simulink model "quadReduced"  (R2024a)
settings: Solver=VariableStepAuto  StartTime=0.0  StopTime=20  RelTol=1e-3
values from neighbouring files (symbols this model uses):
  A_x = 0.25    [playgrounMat.m]    (also in start.m; startEnglPaper.m; startReduced.m)
  A_y = 0.25    [playgrounMat.m]    (also in start.m; startEnglPaper.m; startReduced.m)
  A_z = 0.25    [playgrounMat.m]    (also in start.m; startEnglPaper.m; startReduced.m)
  b = 1.14 * 10^(-7)    (= 1.14e-07)    [start.m]    (also in startEnglPaper.m = 0.033)
  dt = 1e-4    (= 0.0001)    [start.m]    (also in startReduced.m)
  g = 9.81    [playgrounMat.m]    (also in start.m; startEnglPaper.m; startReduced.m)
  gamma_d = pi/3    (= 1.0471975512)    [start.m]    (also in startReduced.m = 0.2)
  I_r = 5.38 * 10 ^ (-5)    (= 5.38e-05)    [start.m]    (also in startEnglPaper.m = 3.38e-05; startReduced.m)
  I_x = 0.0151    [start.m]    (also in startEnglPaper.m = 0.004856; startReduced.m)
  I_y = 0.253    [start.m]    (also in startEnglPaper.m = 0.004856; startReduced.m = 0.0253)
  I_z = 0.0151    [start.m]    (also in startEnglPaper.m = 0.008801; startReduced.m)
  Icm = diag([Ix Iy Iz])    [start.m]    (also in startReduced.m)
  initial_quaternion = quaternion(initial_angles, 'euler', 'ZYX', 'frame')    [start.m]    (also in startReduced.m)
  k = 1.045 * 10^(-11)    (= 1.045e-11)    [start.m]    (also in startEnglPaper.m = 2.98e-06)
  K_gamma_D = 50    [start.m]    (also in startReduced.m = 0.14)
  K_gamma_D1 = K(1)    [playgrounMat.m]    (also in startReduced.m = 0.28992)
  K_gamma_I1 = K(3)    [playgrounMat.m]    (also in startReduced.m = 3.9584)
  K_gamma_P = 108    [start.m]    (also in startReduced.m = 0.35)
  K_gamma_P1 = K(2)    [playgrounMat.m]    (also in startReduced.m = 1.85548)
  K_psi_D = 40    [start.m]    (also in startEnglPaper.m = 9.6; startReduced.m = 0.24)
  K_psi_D1 = 0.0844    [startEnglPaper.m]    (also in startReduced.m = 0.4858)
  K_psi_I1 = 0    [startEnglPaper.m]    (also in startReduced.m = 6.6322)
  K_psi_P = 143    [start.m]    (also in startEnglPaper.m = 23.04; startReduced.m = 0.58)
  K_psi_P1 = 0.202    [startEnglPaper.m]    (also in startReduced.m = 3.11)
  K_theta_D = 58    [start.m]    (also in startEnglPaper.m = 9.6; startReduced.m = 0.14)
  K_theta_P = 141    [start.m]    (also in startEnglPaper.m = 23.04; startReduced.m = 0.35)
  K_y_D = 13.58    [start.m]    (also in startReduced.m)
  K_y_P = 33.18    [start.m]    (also in startReduced.m)
  l = 0.225    [start.m]    (also in startEnglPaper.m; startReduced.m)
  m = 1.44    [playgrounMat.m]    (also in start.m; startEnglPaper.m = 0.486; startReduced.m)
  m_s = [1/4 0 -1/(2*l) -1/(4*a_r); 1/4 -1/(2*l) 0 1/(4*a_r); 1/4 0 1/(2*l) -1/(4*a_r); 1/4 1/(2*l) 0 1/(4*a_r)]    [start.m]    (also in startReduced.m)
  omega_r = 1    [start.m]    (also in startReduced.m = 4)
  P_omega = diag([P_omega_x P_omega_y P_omega_z])    [start.m]    (also in startReduced.m)
  P_q = diag([P_q1 P_q2 P_q3])    [start.m]    (also in startReduced.m)
  psi_d = pi/5    (= 0.628318530718)    [start.m]    (also in startEnglPaper.m = 0.1; startReduced.m = 0.1)
  task_quaternion = quaternion(task_angles, 'euler', 'ZYX', 'frame')    [start.m]    (also in startReduced.m)
  theta_d = pi/4    (= 0.785398163397)    [start.m]    (also in startEnglPaper.m = -0.1; startReduced.m = -0.1)
  y_d = 100    [start.m]    (also in startReduced.m = 0.2)
undefined symbols (not defined in the file or in its folder): compact
libraries: slpidlib x4, aerolibutil x2, sharedtransform x1
(part 1 of 2)
settings Model: Creator=Оздоев  LastModifiedBy=Илья
settings SolverCC: ZeroCrossAlgorithm=Adaptive  AlgebraicLoopSolver=TrustRegion
settings DebuggingCC: IgnoredZcDiagnostic=none  UnconnectedInputMsg=warning  UnconnectedOutputMsg=warning  UnconnectedLineMsg=warning  ArithmeticOperatorsInVariantConditions=warning
settings ModelReferenceCC: EnableRefExpFcnMdlSchedulingChecks=on
settings SFSimCC: CustomCodeUndefinedFunction=UseInterfaceOnly
settings RTWCC: GPUComputeCapability=3.5

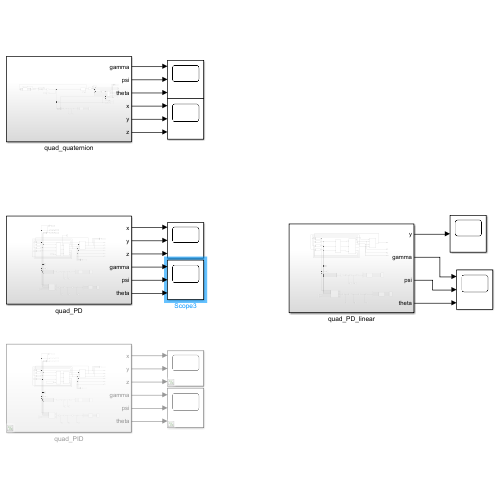
[thumbnail: Simulink's stored preview of the top-level diagram]
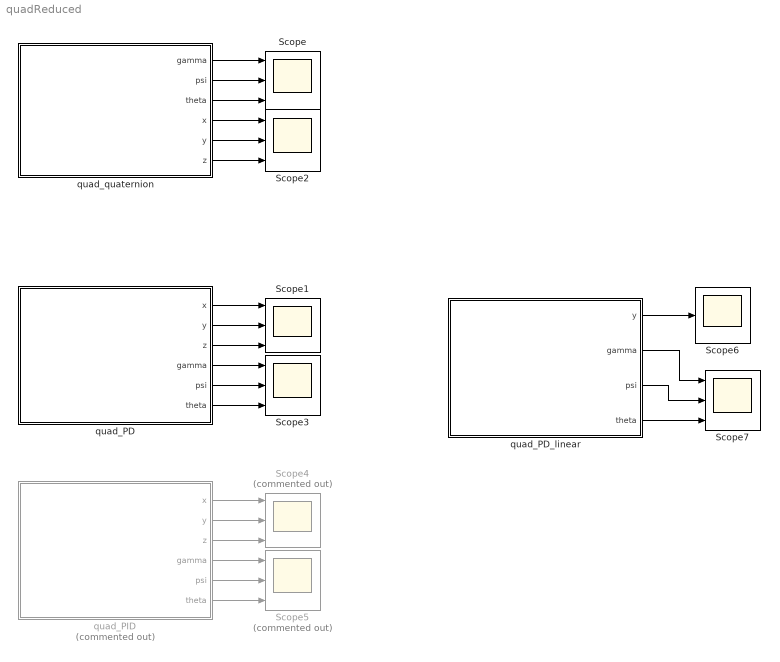
== system quadReduced ==
  Scope{,1..3,7} (5 alike) : Scope  NumInputPorts=3
  Scope4 : Scope  Commented=on  NumInputPorts=3
  Scope5 : Scope  Commented=on  NumInputPorts=3
  Scope6 : Scope
  quad_PD : Subsystem
  quad_PD_linear : Subsystem
  quad_PID : Subsystem  Commented=on
  quad_quaternion : Subsystem
  wires:
  quad_quaternion/1(gamma) -> Scope/1
  quad_quaternion/2(psi) -> Scope/2
  quad_quaternion/3(theta) -> Scope/3
  quad_quaternion/4(x) -> Scope2/1
  quad_quaternion/5(y) -> Scope2/2
  quad_quaternion/6(z) -> Scope2/3
  quad_PD/1(x) -> Scope1/1
  quad_PD/2(y) -> Scope1/2
  quad_PD/3(z) -> Scope1/3
  quad_PD/4(gamma) -> Scope3/1
  quad_PD/5(psi) -> Scope3/2
  quad_PD/6(theta) -> Scope3/3
  quad_PID/6(theta) -> Scope5/3
  quad_PID/5(psi) -> Scope5/2
  quad_PID/4(gamma) -> Scope5/1
  quad_PID/3(z) -> Scope4/3
  quad_PID/2(y) -> Scope4/2
  quad_PID/1(x) -> Scope4/1
  quad_PD_linear/4(theta) -> Scope7/3
  quad_PD_linear/3(psi) -> Scope7/2
  quad_PD_linear/2(gamma) -> Scope7/1
  quad_PD_linear/1(y) -> Scope6/1

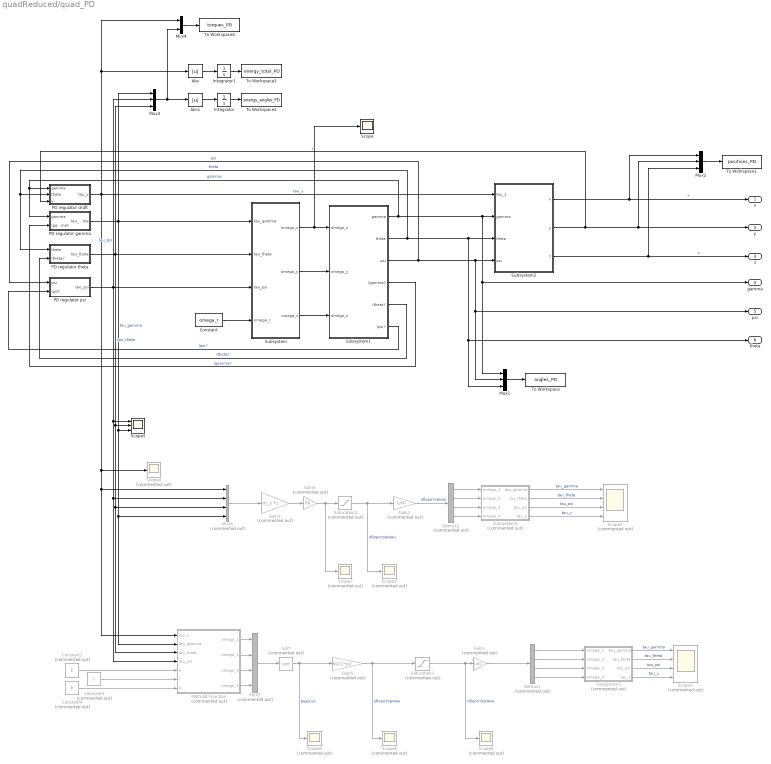
== system quadReduced/quad_PD ==
  Abs : Abs  SaturateOnIntegerOverflow=off
  Abs1 : Abs  SaturateOnIntegerOverflow=off
  Constant : Constant  Value=omega_r
  Constant2 : Constant  Commented=on  Value=k
  Constant3 : Constant  Commented=on  Value=l
  Constant4 : Constant  Commented=on  Value=b
  Demux1 : Demux  Commented=on
  Demux2 : Demux  Commented=on
  Gain1 : Gain  Commented=on  Gain=1/60
  Gain2 : Gain  Commented=on  Gain=1/60
  Gain3 : Gain  Commented=on  Gain=m_s  Multiplication=Matrix(K*u) (u vector)
  Gain5 : Gain  Commented=on  Gain=60/(2*pi)
  Gain6 : Gain  Commented=on  Gain=60
  Integrator : Integrator
  Integrator1 : Integrator
  MATLAB Function : MATLAB Function  Commented=on  TreatAsAtomicUnit=on
  Mux1 : Mux  Inputs=3
  Mux2 : Mux  Inputs=3
  Mux3 : Mux  Inputs=3
  Mux4 : Mux  Inputs=2
  Mux5 : Mux  Commented=on
  Mux6 : Mux  Commented=on
  PD regulator draft : Subsystem
  PD regulator gamma : Subsystem
  PD regulator psi : Subsystem
  PD regulator theta : Subsystem
  Saturation1 : Saturate  Commented=on  UpperLimit=15000  LowerLimit=1000
  Saturation2 : Saturate  Commented=on  UpperLimit=15000  LowerLimit=1000
  Scope : Scope
  Scope1 : Scope  Commented=on  NumInputPorts=4
  Scope{2,4,6..9} (6 alike) : Scope  Commented=on
  Scope3 : Scope  Commented=on  NumInputPorts=4
  Scope5 : Scope  NumInputPorts=3
  Sqrt : Sqrt  Commented=on
  Subsystem : Subsystem
  Subsystem1 : Subsystem
  Subsystem2 : Subsystem
  Subsystem3 : Subsystem  Commented=on
  Subsystem4 : Subsystem  Commented=on
  To Workspace : ToWorkspace  VariableName=angles_PD  SaveFormat=Structure With Time  SampleTime=-1
  To Workspace1 : ToWorkspace  VariableName=positions_PD  SaveFormat=Structure With Time  SampleTime=-1
  To Workspace2 : ToWorkspace  VariableName=energy_angles_PD  SaveFormat=Structure With Time  SampleTime=-1
  To Workspace3 : ToWorkspace  VariableName=energy_total_PD  SaveFormat=Structure With Time  SampleTime=-1
  To Workspace4 : ToWorkspace  VariableName=torques_PD  SaveFormat=Structure With Time  SampleTime=-1
  x : Outport
  y : Outport  Port=2
  z : Outport  Port=3
  gamma : Outport  Port=4
  psi : Outport  Port=5
  theta : Outport  Port=6
  wires:
  Subsystem1/1(gamma) -> gamma/1, Mux1/1, Subsystem2/2(gamma), PD regulator gamma/1(gamma), PD regulator draft/1(gamma)  "gamma"
  Subsystem/2(omega_y) -> Subsystem1/2(omega_y)
  Subsystem/3(omega_z) -> Subsystem1/3(omega_z)
  PD regulator theta/1(tau_theta) -> Subsystem/2(tau_theta), MATLAB Function/3(tau_theta), Mux6/3, Scope5/2, Mux3/3  "tau_theta"
  Mux1/1 -> To Workspace/1
  Subsystem1/5((theta)') -> PD regulator theta/2((theta)')  "(theta)'"
  Constant/1 -> Subsystem/4(omega_r)
  Subsystem/1(omega_x) -> Scope/1, Subsystem1/1(omega_x)
  Subsystem2/1(x) -> Mux2/1, x/1  "x"
  PD regulator gamma/1(tau_gamma) -> Subsystem/1(tau_gamma), Mux3/1, MATLAB Function/2(tau_gamma), Mux6/4, Scope5/3  "tau_gamma"
  Subsystem2/2(y) -> Mux2/2, y/1, PD regulator draft/3(y)  "y"
  Subsystem1/4((gamma)') -> PD regulator gamma/2((gamma)')  "(gamma)'"
  PD regulator psi/1(tau_psi) -> Subsystem/3(tau_psi), Mux3/2, MATLAB Function/4(tau_psi), Mux6/2, Scope5/1  "tau_psi"
  Subsystem1/3(psi) -> psi/1, Mux1/2, Subsystem2/4(psi), PD regulator psi/1(psi)  "psi"
  Subsystem1/6((psi)') -> PD regulator psi/2((psi)')  "(psi)'"
  Subsystem1/2(theta) -> Subsystem2/3(theta), theta/1, Mux1/3, PD regulator theta/1(theta), PD regulator draft/2(theta)  "theta"
  Subsystem2/3(z) -> Mux2/3, z/1  "z"
  Mux2/1 -> To Workspace1/1
  Integrator/1 -> To Workspace2/1
  Mux3/1 -> Mux4/2, Abs1/1
  Integrator1/1 -> To Workspace3/1
  Abs/1 -> Integrator1/1
  Abs1/1 -> Integrator/1
  Mux4/1 -> To Workspace4/1
  Subsystem3/2(tau_theta) -> Scope1/2  "tau_theta"
  Subsystem3/3(tau_psi) -> Scope1/3  "tau_psi"
  Subsystem3/1(tau_gamma) -> Scope1/1  "tau_gamma"
  Constant2/1 -> MATLAB Function/5(k)
  Constant3/1 -> MATLAB Function/6(l)
  Constant4/1 -> MATLAB Function/7(b)
  MATLAB Function/1(omega_1) -> Mux5/1
  MATLAB Function/2(omega_2) -> Mux5/2
  MATLAB Function/3(omega_3) -> Mux5/3
  MATLAB Function/4(omega_4) -> Mux5/4
  Mux5/1 -> Sqrt/1
  PD regulator draft/1(tau_y) -> Subsystem2/1(tau_y), Abs/1, Mux4/1, MATLAB Function/1(tau_y), Mux6/1, Scope4/1  "tau_y"
  Subsystem3/4(tau_y) -> Scope1/4  "tau_y"
  Mux6/1 -> Gain3/1
  Subsystem4/2(tau_theta) -> Scope3/2  "tau_theta"
  Subsystem4/3(tau_psi) -> Scope3/3  "tau_psi"
  Demux2/2 -> Subsystem4/2(omega_2)
  Demux2/1 -> Subsystem4/1(omega_1)
  Demux2/4 -> Subsystem4/4(omega_4)
  Demux2/3 -> Subsystem4/3(omega_3)
  Subsystem4/4(tau_y) -> Scope3/4  "tau_y"
  Subsystem4/1(tau_gamma) -> Scope3/1  "tau_gamma"
  Demux1/3 -> Subsystem3/3(omega_3)
  Demux1/4 -> Subsystem3/4(omega_4)
  Demux1/1 -> Subsystem3/1(omega_1)
  Demux1/2 -> Subsystem3/2(omega_2)
  Saturation2/1 -> Gain2/1, Scope2/1  "оборотов/мин"
  Gain6/1 -> Scope7/1, Saturation2/1
  Sqrt/1 -> Scope9/1, Gain5/1  "рад/сек"
  Saturation1/1 -> Gain1/1, Scope6/1  "оборотов/мин"
  Gain3/1 -> Gain6/1
  Gain5/1 -> Saturation1/1, Scope8/1  "оборотов/мин"
  Gain1/1 -> Demux1/1
  Gain2/1 -> Demux2/1  "оборотов/сек"

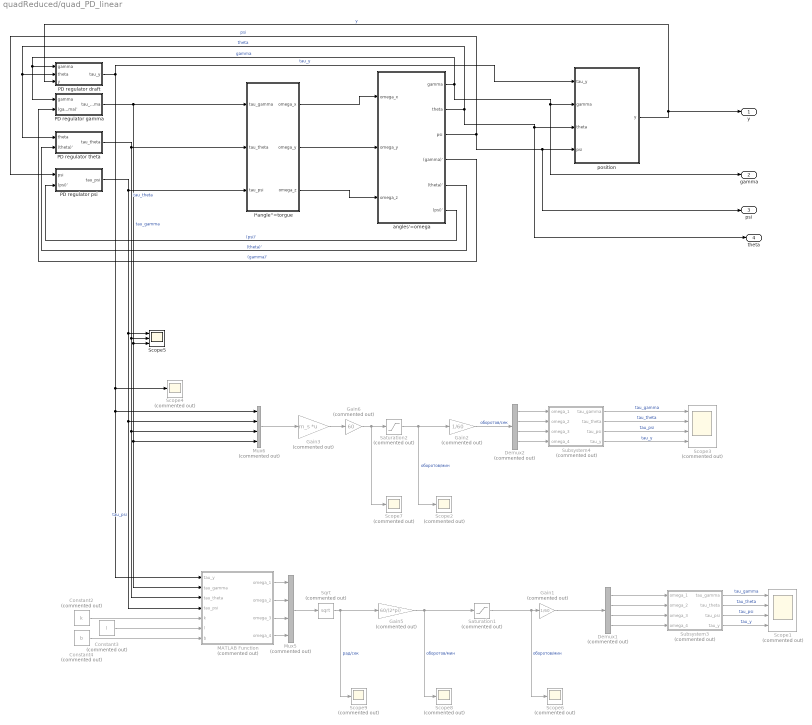
== system quadReduced/quad_PD_linear ==
  Constant2 : Constant  Commented=on  Value=k
  Constant3 : Constant  Commented=on  Value=l
  Constant4 : Constant  Commented=on  Value=b
  Demux1 : Demux  Commented=on
  Demux2 : Demux  Commented=on
  Gain1 : Gain  Commented=on  Gain=1/60
  Gain2 : Gain  Commented=on  Gain=1/60
  Gain3 : Gain  Commented=on  Gain=m_s  Multiplication=Matrix(K*u) (u vector)
  Gain5 : Gain  Commented=on  Gain=60/(2*pi)
  Gain6 : Gain  Commented=on  Gain=60
  I*angle''=torgue : Subsystem
  MATLAB Function : MATLAB Function  Commented=on  TreatAsAtomicUnit=on
  Mux5 : Mux  Commented=on
  Mux6 : Mux  Commented=on
  PD regulator draft : Subsystem
  PD regulator gamma : Subsystem
  PD regulator psi : Subsystem
  PD regulator theta : Subsystem
  Saturation1 : Saturate  Commented=on  UpperLimit=15000  LowerLimit=1000
  Saturation2 : Saturate  Commented=on  UpperLimit=15000  LowerLimit=1000
  Scope1 : Scope  Commented=on  NumInputPorts=4
  Scope{2,4,6..9} (6 alike) : Scope  Commented=on
  Scope3 : Scope  Commented=on  NumInputPorts=4
  Scope5 : Scope  NumInputPorts=3
  Sqrt : Sqrt  Commented=on
  Subsystem3 : Subsystem  Commented=on
  Subsystem4 : Subsystem  Commented=on
  angles'=omega : Subsystem
  position : Subsystem
  y : Outport
  gamma : Outport  Port=2
  psi : Outport  Port=3
  theta : Outport  Port=4
  wires:
  Gain2/1 -> Demux2/1  "оборотов/сек"
  Gain1/1 -> Demux1/1
  Gain5/1 -> Scope8/1, Saturation1/1  "оборотов/мин"
  Gain3/1 -> Gain6/1
  Saturation1/1 -> Scope6/1, Gain1/1  "оборотов/мин"
  Sqrt/1 -> Gain5/1, Scope9/1  "рад/сек"
  Gain6/1 -> Saturation2/1, Scope7/1
  Saturation2/1 -> Scope2/1, Gain2/1  "оборотов/мин"
  Demux1/2 -> Subsystem3/2(omega_2)
  Demux1/1 -> Subsystem3/1(omega_1)
  Demux1/4 -> Subsystem3/4(omega_4)
  Demux1/3 -> Subsystem3/3(omega_3)
  Subsystem4/1(tau_gamma) -> Scope3/1  "tau_gamma"
  Subsystem4/4(tau_y) -> Scope3/4  "tau_y"
  Demux2/3 -> Subsystem4/3(omega_3)
  Demux2/4 -> Subsystem4/4(omega_4)
  Demux2/1 -> Subsystem4/1(omega_1)
  Demux2/2 -> Subsystem4/2(omega_2)
  Subsystem4/3(tau_psi) -> Scope3/3  "tau_psi"
  Subsystem4/2(tau_theta) -> Scope3/2  "tau_theta"
  Mux6/1 -> Gain3/1
  Subsystem3/4(tau_y) -> Scope1/4  "tau_y"
  PD regulator draft/1(tau_y) -> Scope4/1, Mux6/1, MATLAB Function/1(tau_y), position/1(tau_y)  "tau_y"
  Mux5/1 -> Sqrt/1
  MATLAB Function/4(omega_4) -> Mux5/4
  MATLAB Function/3(omega_3) -> Mux5/3
  MATLAB Function/2(omega_2) -> Mux5/2
  MATLAB Function/1(omega_1) -> Mux5/1
  Constant4/1 -> MATLAB Function/7(b)
  Constant3/1 -> MATLAB Function/6(l)
  Constant2/1 -> MATLAB Function/5(k)
  Subsystem3/1(tau_gamma) -> Scope1/1  "tau_gamma"
  Subsystem3/3(tau_psi) -> Scope1/3  "tau_psi"
  Subsystem3/2(tau_theta) -> Scope1/2  "tau_theta"
  angles'=omega/2(theta) -> theta/1, position/3(theta), PD regulator draft/2(theta), PD regulator theta/1(theta)  "theta"
  angles'=omega/6((psi)') -> PD regulator psi/2((psi)')  "(psi)'"
  angles'=omega/3(psi) -> position/4(psi), psi/1, PD regulator psi/1(psi)  "psi"
  PD regulator psi/1(tau_psi) -> Scope5/1, Mux6/2, MATLAB Function/4(tau_psi), I*angle''=torgue/3(tau_psi)  "tau_psi"
  angles'=omega/4((gamma)') -> PD regulator gamma/2((gamma)')  "(gamma)'"
  position/1(y) -> PD regulator draft/3(y), y/1  "y"
  PD regulator gamma/1(tau_gamma) -> Scope5/3, Mux6/4, MATLAB Function/2(tau_gamma), I*angle''=torgue/1(tau_gamma)  "tau_gamma"
  I*angle''=torgue/1(omega_x) -> angles'=omega/1(omega_x)
  angles'=omega/5((theta)') -> PD regulator theta/2((theta)')  "(theta)'"
  PD regulator theta/1(tau_theta) -> Scope5/2, Mux6/3, MATLAB Function/3(tau_theta), I*angle''=torgue/2(tau_theta)  "tau_theta"
  I*angle''=torgue/3(omega_z) -> angles'=omega/3(omega_z)
  I*angle''=torgue/2(omega_y) -> angles'=omega/2(omega_y)
  angles'=omega/1(gamma) -> gamma/1, position/2(gamma), PD regulator draft/1(gamma), PD regulator gamma/1(gamma)  "gamma"

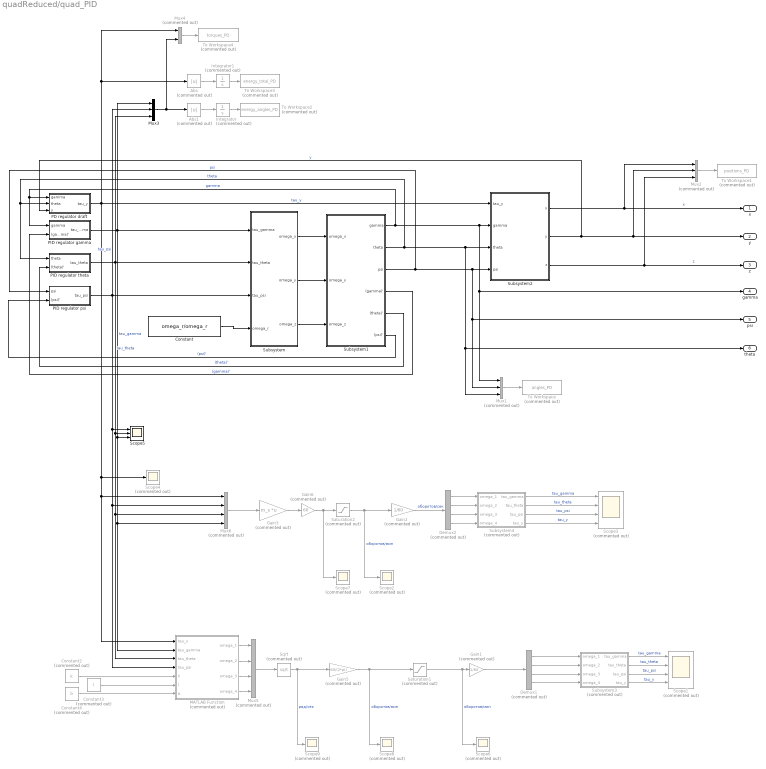
== system quadReduced/quad_PID ==
  Abs : Abs  Commented=on  SaturateOnIntegerOverflow=off
  Abs1 : Abs  Commented=on  SaturateOnIntegerOverflow=off
  Constant : Constant  Value=omega_r/omega_r
  Constant2 : Constant  Commented=on  Value=k
  Constant3 : Constant  Commented=on  Value=l
  Constant4 : Constant  Commented=on  Value=b
  Demux1 : Demux  Commented=on
  Demux2 : Demux  Commented=on
  Gain1 : Gain  Commented=on  Gain=1/60
  Gain2 : Gain  Commented=on  Gain=1/60
  Gain3 : Gain  Commented=on  Gain=m_s  Multiplication=Matrix(K*u) (u vector)
  Gain5 : Gain  Commented=on  Gain=60/(2*pi)
  Gain6 : Gain  Commented=on  Gain=60
  Integrator : Integrator  Commented=on
  Integrator1 : Integrator  Commented=on
  MATLAB Function : MATLAB Function  Commented=on  TreatAsAtomicUnit=on
  Mux1 : Mux  Commented=on  Inputs=3
  Mux2 : Mux  Commented=on  Inputs=3
  Mux3 : Mux  Inputs=3
  Mux4 : Mux  Commented=on  Inputs=2
  Mux5 : Mux  Commented=on
  Mux6 : Mux  Commented=on
  PD regulator draft : Subsystem
  PID regulator gamma : Subsystem
  PID regulator psi : Subsystem
  PID regulator theta : Subsystem
  Saturation1 : Saturate  Commented=on  UpperLimit=15000  LowerLimit=1000
  Saturation2 : Saturate  Commented=on  UpperLimit=15000  LowerLimit=1000
  Scope1 : Scope  Commented=on  NumInputPorts=4
  Scope{2,4,6..9} (6 alike) : Scope  Commented=on
  Scope3 : Scope  Commented=on  NumInputPorts=4
  Scope5 : Scope  NumInputPorts=3
  Sqrt : Sqrt  Commented=on
  Subsystem : Subsystem
  Subsystem1 : Subsystem
  Subsystem2 : Subsystem
  Subsystem3 : Subsystem  Commented=on
  Subsystem4 : Subsystem  Commented=on
  To Workspace : ToWorkspace  Commented=on  VariableName=angles_PD  SaveFormat=Structure With Time  SampleTime=-1
  To Workspace1 : ToWorkspace  Commented=on  VariableName=positions_PD  SaveFormat=Structure With Time  SampleTime=-1
  To Workspace2 : ToWorkspace  Commented=on  VariableName=energy_angles_PD  SaveFormat=Structure With Time  SampleTime=-1
  To Workspace3 : ToWorkspace  Commented=on  VariableName=energy_total_PD  SaveFormat=Structure With Time  SampleTime=-1
  To Workspace4 : ToWorkspace  Commented=on  VariableName=torques_PD  SaveFormat=Structure With Time  SampleTime=-1
  x : Outport
  y : Outport  Port=2
  z : Outport  Port=3
  gamma : Outport  Port=4
  psi : Outport  Port=5
  theta : Outport  Port=6
  wires:
  Gain2/1 -> Demux2/1  "оборотов/сек"
  Gain1/1 -> Demux1/1
  Gain5/1 -> Scope8/1, Saturation1/1  "оборотов/мин"
  Gain3/1 -> Gain6/1
  Saturation1/1 -> Scope6/1, Gain1/1  "оборотов/мин"
  Sqrt/1 -> Gain5/1, Scope9/1  "рад/сек"
  Gain6/1 -> Saturation2/1, Scope7/1
  Saturation2/1 -> Scope2/1, Gain2/1  "оборотов/мин"
  Demux1/2 -> Subsystem3/2(omega_2)
  Demux1/1 -> Subsystem3/1(omega_1)
  Demux1/4 -> Subsystem3/4(omega_4)
  Demux1/3 -> Subsystem3/3(omega_3)
  Subsystem4/1(tau_gamma) -> Scope3/1  "tau_gamma"
  Subsystem4/4(tau_y) -> Scope3/4  "tau_y"
  Demux2/3 -> Subsystem4/3(omega_3)
  Demux2/4 -> Subsystem4/4(omega_4)
  Demux2/1 -> Subsystem4/1(omega_1)
  Demux2/2 -> Subsystem4/2(omega_2)
  Subsystem4/3(tau_psi) -> Scope3/3  "tau_psi"
  Subsystem4/2(tau_theta) -> Scope3/2  "tau_theta"
  Mux6/1 -> Gain3/1
  Subsystem3/4(tau_y) -> Scope1/4  "tau_y"
  PD regulator draft/1(tau_y) -> Scope4/1, Mux6/1, MATLAB Function/1(tau_y), Mux4/1, Abs/1, Subsystem2/1(tau_y)  "tau_y"
  Mux5/1 -> Sqrt/1
  MATLAB Function/4(omega_4) -> Mux5/4
  MATLAB Function/3(omega_3) -> Mux5/3
  MATLAB Function/2(omega_2) -> Mux5/2
  MATLAB Function/1(omega_1) -> Mux5/1
  Constant4/1 -> MATLAB Function/7(b)
  Constant3/1 -> MATLAB Function/6(l)
  Constant2/1 -> MATLAB Function/5(k)
  Subsystem3/1(tau_gamma) -> Scope1/1  "tau_gamma"
  Subsystem3/3(tau_psi) -> Scope1/3  "tau_psi"
  Subsystem3/2(tau_theta) -> Scope1/2  "tau_theta"
  Mux4/1 -> To Workspace4/1
  Abs1/1 -> Integrator/1
  Abs/1 -> Integrator1/1
  Integrator1/1 -> To Workspace3/1
  Mux3/1 -> Abs1/1, Mux4/2
  Integrator/1 -> To Workspace2/1
  Mux2/1 -> To Workspace1/1
  Subsystem2/3(z) -> z/1, Mux2/3  "z"
  Subsystem1/2(theta) -> PD regulator draft/2(theta), PID regulator theta/1(theta), Mux1/3, theta/1, Subsystem2/3(theta)  "theta"
  Subsystem1/6((psi)') -> PID regulator psi/2((psi)')  "(psi)'"
  Subsystem1/3(psi) -> PID regulator psi/1(psi), Subsystem2/4(psi), Mux1/2, psi/1  "psi"
  PID regulator psi/1(tau_psi) -> Scope5/1, Mux6/2, MATLAB Function/4(tau_psi), Mux3/2, Subsystem/3(tau_psi)  "tau_psi"
  Subsystem1/4((gamma)') -> PID regulator gamma/2((gamma)')  "(gamma)'"
  Subsystem2/2(y) -> PD regulator draft/3(y), y/1, Mux2/2  "y"
  PID regulator gamma/1(tau_gamma) -> Scope5/3, Mux6/4, MATLAB Function/2(tau_gamma), Mux3/1, Subsystem/1(tau_gamma)  "tau_gamma"
  Subsystem2/1(x) -> x/1, Mux2/1  "x"
  Subsystem/1(omega_x) -> Subsystem1/1(omega_x)
  Constant/1 -> Subsystem/4(omega_r)
  Subsystem1/5((theta)') -> PID regulator theta/2((theta)')  "(theta)'"
  Mux1/1 -> To Workspace/1
  PID regulator theta/1(tau_theta) -> Mux3/3, Scope5/2, Mux6/3, MATLAB Function/3(tau_theta), Subsystem/2(tau_theta)  "tau_theta"
  Subsystem/3(omega_z) -> Subsystem1/3(omega_z)
  Subsystem/2(omega_y) -> Subsystem1/2(omega_y)
  Subsystem1/1(gamma) -> PD regulator draft/1(gamma), PID regulator gamma/1(gamma), Subsystem2/2(gamma), Mux1/1, gamma/1  "gamma"

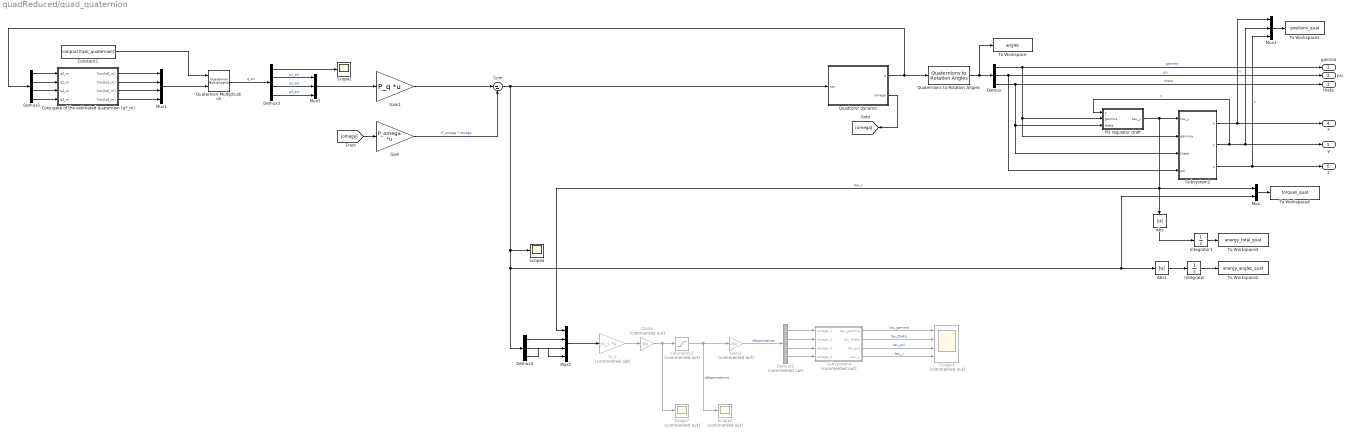
== system quadReduced/quad_quaternion ==
  " Сonjugate of the estimated quaternion (q*_m)" : Subsystem
  Abs : Abs  SaturateOnIntegerOverflow=off
  Abs1 : Abs  SaturateOnIntegerOverflow=off
  Constant1 : Constant  Value=compact(task_quaternion)'
  Demux : Demux  Outputs=3
  Demux1 : Demux
  Demux2 : Demux  Commented=on
  Demux3 : Demux
  Demux4 : Demux  Outputs=3
  Gain : Gain  Gain=P_omega  Multiplication=Matrix(K*u) (u vector)
  Gain1 : Gain  Gain=P_q  Multiplication=Matrix(K*u) (u vector)
  Gain2 : Gain  Commented=on  Gain=1/60
  Gain6 : Gain  Commented=on  Gain=60
  Integrator : Integrator
  Integrator1 : Integrator
  Mux : Mux  Inputs=2
  Mux1 : Mux
  Mux2 : Mux
  Mux3 : Mux  Inputs=3
  Mux5 : Mux  Inputs=3
  PD regulator draft : Subsystem
  Quadtoror dynamic : Subsystem
  Quaternion Multiplication : aerolibutil/Quaternion Multiplication
  Quaternions to Rotation Angles : sharedtransform/Quaternions to Rotation Angles  rotationOrder=ZYX  aMode=aMode
  Saturation2 : Saturate  Commented=on  UpperLimit=15000  LowerLimit=1000
  Scope1 : Scope
  Scope2 : Scope  Commented=on
  Scope3 : Scope  Commented=on  NumInputPorts=4
  Scope4 : Scope
  Scope7 : Scope  Commented=on
  Subsystem2 : Subsystem
  Subsystem4 : Subsystem  Commented=on
  Sum : Sum  Inputs=|--
  To Workspace : ToWorkspace  VariableName=angles  SaveFormat=Structure With Time  SampleTime=-1
  To Workspace1 : ToWorkspace  VariableName=positions_quat  SaveFormat=Structure With Time  SampleTime=-1
  To Workspace2 : ToWorkspace  VariableName=energy_angles_quat  SaveFormat=Structure With Time  SampleTime=-1
  To Workspace3 : ToWorkspace  VariableName=energy_total_quat  SaveFormat=Structure With Time  SampleTime=-1
  To Workspace4 : ToWorkspace  VariableName=torques_quat  SaveFormat=Structure With Time  SampleTime=-1
  m_s : Gain  Commented=on  Gain=m_s  Multiplication=Matrix(K*u) (u vector)
  gamma : Outport
  psi : Outport  Port=2
  theta : Outport  Port=3
  x : Outport  Port=4
  y : Outport  Port=5
  z : Outport  Port=6
  wires:
  Demux3/2 -> Mux5/1  "q1_err"
  Mux1/1 -> Quaternion Multiplication/2
  Demux/3 -> theta/1, PD regulator draft/3(theta), Subsystem2/3(theta)  "theta"
  Demux1/1 -> " Сonjugate of the estimated quaternion (q*_m)"/1(q0_m)
  " Сonjugate of the estimated quaternion (q*_m)"/4(Conj(q3_m)) -> Mux1/4
  Demux1/4 -> " Сonjugate of the estimated quaternion (q*_m)"/4(q3_m)
  Quadtoror dynamic/1(q) -> Demux1/1, Quaternions to Rotation Angles/1
  " Сonjugate of the estimated quaternion (q*_m)"/2(Conj(q1_m)) -> Mux1/2
  Quaternions to Rotation Angles/1 -> Demux/1, To Workspace/1
  Subsystem2/2(y) -> Mux3/2, y/1, PD regulator draft/1(y)  "y"
  " Сonjugate of the estimated quaternion (q*_m)"/3(Conj(q2_m)) -> Mux1/3
  Demux/1 -> gamma/1, Subsystem2/2(gamma), PD regulator draft/2(gamma)  "gamma"
  Quadtoror dynamic/2(omega) -> [omega]
  Demux3/3 -> Mux5/2  "q2_err"
  Demux/2 -> psi/1, Subsystem2/4(psi)  "psi"
  " Сonjugate of the estimated quaternion (q*_m)"/1(Conj(q0_m)) -> Mux1/1
  Mux5/1 -> Gain1/1
  Demux3/1 -> Scope1/1
  [omega] -> Gain/1
  Demux3/4 -> Mux5/3  "q3_err"
  Constant1/1 -> Quaternion Multiplication/1
  Demux1/3 -> " Сonjugate of the estimated quaternion (q*_m)"/3(q2_m)
  Gain1/1 -> Sum/1
  PD regulator draft/1(tau_y) -> Subsystem2/1(tau_y), Mux2/1, Mux/1, Abs/1  "tau_y"
  Demux1/2 -> " Сonjugate of the estimated quaternion (q*_m)"/2(q1_m)
  Quaternion Multiplication/1 -> Demux3/1  "q_err"
  Gain/1 -> Sum/2  "P_omega * omega"
  Subsystem2/3(z) -> Mux3/3, z/1  "z"
  Subsystem2/1(x) -> Mux3/1, x/1  "x"
  Mux3/1 -> To Workspace1/1
  Integrator1/1 -> To Workspace3/1
  Integrator/1 -> To Workspace2/1
  Abs/1 -> Integrator1/1
  Abs1/1 -> Integrator/1
  Mux/1 -> To Workspace4/1
  Subsystem4/3(tau_psi) -> Scope3/3  "tau_psi"
  Saturation2/1 -> Gain2/1, Scope2/1  "оборотов/мин"
  Gain6/1 -> Scope7/1, Saturation2/1
  Subsystem4/4(tau_y) -> Scope3/4  "tau_y"
  Demux2/2 -> Subsystem4/2(omega_2)
  Subsystem4/1(tau_gamma) -> Scope3/1  "tau_gamma"
  Demux2/4 -> Subsystem4/4(omega_4)
  Demux2/3 -> Subsystem4/3(omega_3)
  Demux2/1 -> Subsystem4/1(omega_1)
  m_s/1 -> Gain6/1
  Subsystem4/2(tau_theta) -> Scope3/2  "tau_theta"
  Gain2/1 -> Demux2/1  "оборотов/сек"
  Demux4/3 -> Mux2/3
  Mux2/1 -> m_s/1
  Sum/1 -> Quadtoror dynamic/1(tau), Scope4/1, Demux4/1, Mux/2, Abs1/1
  Demux4/2 -> Mux2/4
  Demux4/1 -> Mux2/2

== system quadReduced/quad_PD/PD regulator draft ==
  gamma : Inport
  theta : Inport  Port=2
  y : Inport  Port=3
  Constant : Constant  Value=g
  Constant1 : Constant  Value=K_y_D
  Constant4 : Constant  Value=K_y_P
  Constant7 : Constant  Value=m
  Cos : Trigonometry  Operator=cos
  Cos1 : Trigonometry  Operator=cos
  Derivative : Derivative
  Derivative1 : Derivative
  Product{,1,3..4} (4 alike) : Product
  Product2 : Product  Inputs=*/
  Sum : Sum  Inputs=+++
  Sum1 : Sum  Inputs=|+-
  Sum2 : Sum  Inputs=|+-
  target : Constant  Value=y_d
  target1 : Constant  Value=y_d
  tau_y : Outport
  wires:
  Cos/1 -> Product3/1
  Product/1 -> Sum/1
  Constant1/1 -> Product/1
  Product1/1 -> Sum/3
  Sum1/1 -> Product/2
  Constant4/1 -> Product1/1
  target/1 -> Derivative/1
  y/1 -> Sum2/2, Derivative1/1  "y"
  Derivative1/1 -> Sum1/2
  Constant/1 -> Sum/2
  Derivative/1 -> Sum1/1
  target1/1 -> Sum2/1
  Product3/1 -> Product2/2
  Constant7/1 -> Product2/1
  Cos1/1 -> Product3/2
  Sum2/1 -> Product1/2
  theta/1 -> Cos1/1  "theta"
  gamma/1 -> Cos/1  "gamma"
  Sum/1 -> Product4/1
  Product4/1 -> tau_y/1  "tau_y"
  Product2/1 -> Product4/2

== system quadReduced/quad_PD/PD regulator gamma ==
  gamma : Inport
  (gamma)' : Inport  Port=2
  Constant : Constant  Value=I_x/I_x
  Constant1 : Constant  Value=K_gamma_D
  Constant2 : Constant  Value=gamma_d
  Constant4 : Constant  Value=K_gamma_P
  Constant5 : Constant  Value=gamma_d
  Derivative : Derivative
  Product : Product
  Product1 : Product
  Product2 : Product
  Sum : Sum  Inputs=++|
  Sum1 : Sum  Inputs=|+-
  Sum2 : Sum  Inputs=|+-
  tau_gamma : Outport
  wires:
  Product/1 -> Sum/1
  Constant1/1 -> Product/1
  Product1/1 -> Sum/2
  Sum1/1 -> Product/2
  Constant4/1 -> Product1/1
  gamma/1 -> Sum2/2
  Constant5/1 -> Sum2/1
  Derivative/1 -> Sum1/1
  Constant2/1 -> Derivative/1
  (gamma)'/1 -> Sum1/2
  Sum2/1 -> Product1/2
  Product2/1 -> tau_gamma/1  "tau_gamma"
  Constant/1 -> Product2/2
  Sum/1 -> Product2/1

== system quadReduced/quad_PD/PD regulator psi ==
  psi : Inport
  (psi)' : Inport  Port=2
  Constant : Constant  Value=I_y/I_y
  Constant1 : Constant  Value=K_psi_D
  Constant2 : Constant  Value=psi_d
  Constant4 : Constant  Value=K_psi_P
  Constant5 : Constant  Value=psi_d
  Derivative : Derivative
  Product : Product
  Product1 : Product
  Product2 : Product
  Sum : Sum  Inputs=++|
  Sum1 : Sum  Inputs=|+-
  Sum2 : Sum  Inputs=|+-
  tau_psi : Outport
  wires:
  Product/1 -> Sum/1
  Constant1/1 -> Product/1
  Product1/1 -> Sum/2
  Sum1/1 -> Product/2
  Constant4/1 -> Product1/1
  psi/1 -> Sum2/2
  Constant5/1 -> Sum2/1
  Derivative/1 -> Sum1/1
  Constant2/1 -> Derivative/1
  (psi)'/1 -> Sum1/2
  Sum2/1 -> Product1/2
  Product2/1 -> tau_psi/1  "tau_psi"
  Constant/1 -> Product2/2
  Sum/1 -> Product2/1

== system quadReduced/quad_PD/PD regulator theta ==
  theta : Inport
  (theta)' : Inport  Port=2
  Constant : Constant  Value=I_z/I_z
  Constant1 : Constant  Value=K_theta_D
  Constant2 : Constant  Value=theta_d
  Constant4 : Constant  Value=K_theta_P
  Constant5 : Constant  Value=theta_d
  Derivative : Derivative
  Product : Product
  Product1 : Product
  Product2 : Product
  Sum : Sum  Inputs=++|
  Sum1 : Sum  Inputs=|+-
  Sum2 : Sum  Inputs=|+-
  tau_theta : Outport
  wires:
  Product/1 -> Sum/1
  Constant1/1 -> Product/1
  Product1/1 -> Sum/2
  Sum1/1 -> Product/2
  Constant4/1 -> Product1/1
  theta/1 -> Sum2/2
  Constant5/1 -> Sum2/1
  Derivative/1 -> Sum1/1
  Constant2/1 -> Derivative/1
  (theta)'/1 -> Sum1/2
  Sum2/1 -> Product1/2
  Product2/1 -> tau_theta/1  "tau_theta"
  Constant/1 -> Product2/2
  Sum/1 -> Product2/1

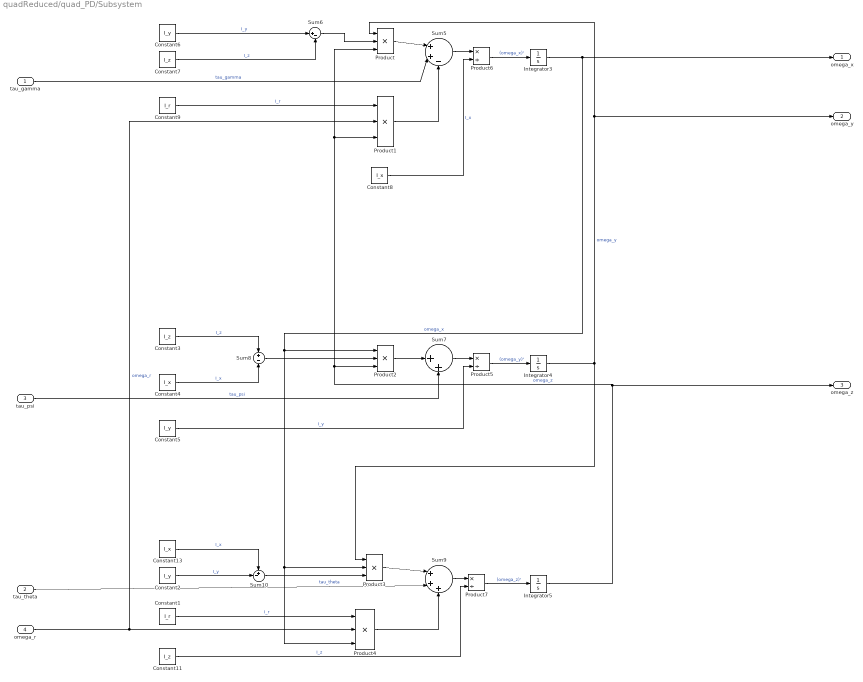
== system quadReduced/quad_PD/Subsystem ==
  tau_gamma : Inport
  tau_theta : Inport  Port=2
  tau_psi : Inport  Port=3
  omega_r : Inport  Port=4
  Constant1 : Constant  Value=I_r
  Constant11 : Constant  Value=I_z
  Constant13 : Constant  Value=I_x
  Constant2 : Constant  Value=I_y
  Constant3 : Constant  Value=I_z
  Constant4 : Constant  Value=I_x
  Constant5 : Constant  Value=I_y
  Constant6 : Constant  Value=I_y
  Constant7 : Constant  Value=I_z
  Constant8 : Constant  Value=I_x
  Constant9 : Constant  Value=I_r
  Integrator3 : Integrator
  Integrator4 : Integrator
  Integrator5 : Integrator
  Product{,1..4} (5 alike) : Product  Inputs=3
  Product5 : Product  Inputs=*/
  Product6 : Product  Inputs=*/
  Product7 : Product  Inputs=*/
  Sum10 : Sum  Inputs=+-|
  Sum5 : Sum  Inputs=|++-
  Sum6 : Sum  Inputs=|+-
  Sum7 : Sum  Inputs=|++
  Sum8 : Sum  Inputs=+|-
  Sum9 : Sum  Inputs=|+++
  omega_x : Outport
  omega_y : Outport  Port=2
  omega_z : Outport  Port=3
  wires:
  Integrator5/1 -> Product2/3, Product/3, Product1/3, omega_z/1  "omega_z"
  Constant13/1 -> Sum10/1  "I_x"
  Integrator3/1 -> omega_x/1, Product4/3, Product3/2, Product2/1  "omega_x"
  Product1/1 -> Sum5/3
  Product/1 -> Sum5/1
  Sum10/1 -> Product3/3
  tau_psi/1 -> Sum7/2  "tau_psi"
  Constant7/1 -> Sum6/2  "I_z"
  Integrator4/1 -> omega_y/1, Product/1, Product3/1  "omega_y"
  omega_r/1 -> Product4/2, Product1/2  "omega_r"
  Product2/1 -> Sum7/1
  Sum5/1 -> Product6/1
  Constant9/1 -> Product1/1  "I_r"
  Constant6/1 -> Sum6/1  "I_y"
  Sum8/1 -> Product2/2
  Sum7/1 -> Product5/1
  Sum6/1 -> Product/2
  Product6/1 -> Integrator3/1  "(omega_x)'"
  Product3/1 -> Sum9/1
  Sum9/1 -> Product7/1
  Product4/1 -> Sum9/3
  Product5/1 -> Integrator4/1  "(omega_y)'"
  Product7/1 -> Integrator5/1  "(omega_z)'"
  tau_gamma/1 -> Sum5/2  "tau_gamma"
  tau_theta/1 -> Sum9/2  "tau_theta"
  Constant1/1 -> Product4/1  "I_r"
  Constant2/1 -> Sum10/2  "I_y"
  Constant3/1 -> Sum8/1  "I_z"
  Constant4/1 -> Sum8/2  "I_x"
  Constant5/1 -> Product5/2  "I_y"
  Constant8/1 -> Product6/2  "I_x"
  Constant11/1 -> Product7/2  "I_z"

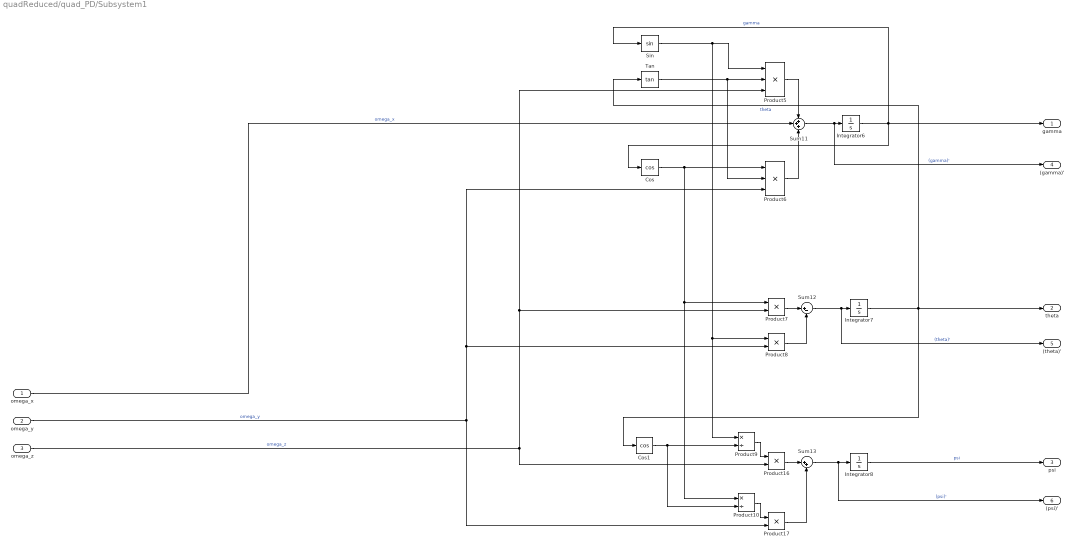
== system quadReduced/quad_PD/Subsystem1 ==
  omega_x : Inport
  omega_y : Inport  Port=2
  omega_z : Inport  Port=3
  Cos : Trigonometry  Operator=cos
  Cos1 : Trigonometry  Operator=cos
  Integrator6 : Integrator
  Integrator7 : Integrator
  Integrator8 : Integrator
  Product10 : Product  Inputs=*/
  Product{7..8,16..17} (4 alike) : Product
  Product5 : Product  Inputs=3
  Product6 : Product  Inputs=3
  Product9 : Product  Inputs=*/
  Sin : Trigonometry
  Sum11 : Sum  Inputs=+++
  Sum12 : Sum  Inputs=|+-
  Sum13 : Sum  Inputs=|++
  Tan : Trigonometry  Operator=tan
  gamma : Outport
  theta : Outport  Port=2
  psi : Outport  Port=3
  (gamma)' : Outport  Port=4
  (theta)' : Outport  Port=5
  (psi)' : Outport  Port=6
  wires:
  Product9/1 -> Product16/1
  Sum13/1 -> (psi)'/1, Integrator8/1  "(psi)'"
  omega_x/1 -> Sum11/2  "omega_x"
  Tan/1 -> Product5/2, Product6/2
  Sum11/1 -> (gamma)'/1, Integrator6/1  "(gamma)'"
  Sin/1 -> Product9/1, Product8/1, Product5/1
  Cos1/1 -> Product10/2, Product9/2
  Product16/1 -> Sum13/1
  Integrator7/1 -> theta/1, Tan/1, Cos1/1  "theta"
  Product5/1 -> Sum11/1
  Integrator6/1 -> Cos/1, gamma/1, Sin/1  "gamma"
  Product8/1 -> Sum12/2
  Product7/1 -> Sum12/1
  Cos/1 -> Product10/1, Product7/1, Product6/1
  omega_z/1 -> Product7/2, Product5/3, Product16/2  "omega_z"
  omega_y/1 -> Product6/3, Product8/2, Product17/2  "omega_y"
  Product6/1 -> Sum11/3
  Integrator8/1 -> psi/1  "psi"
  Sum12/1 -> (theta)'/1, Integrator7/1  "(theta)'"
  Product10/1 -> Product17/1
  Product17/1 -> Sum13/2

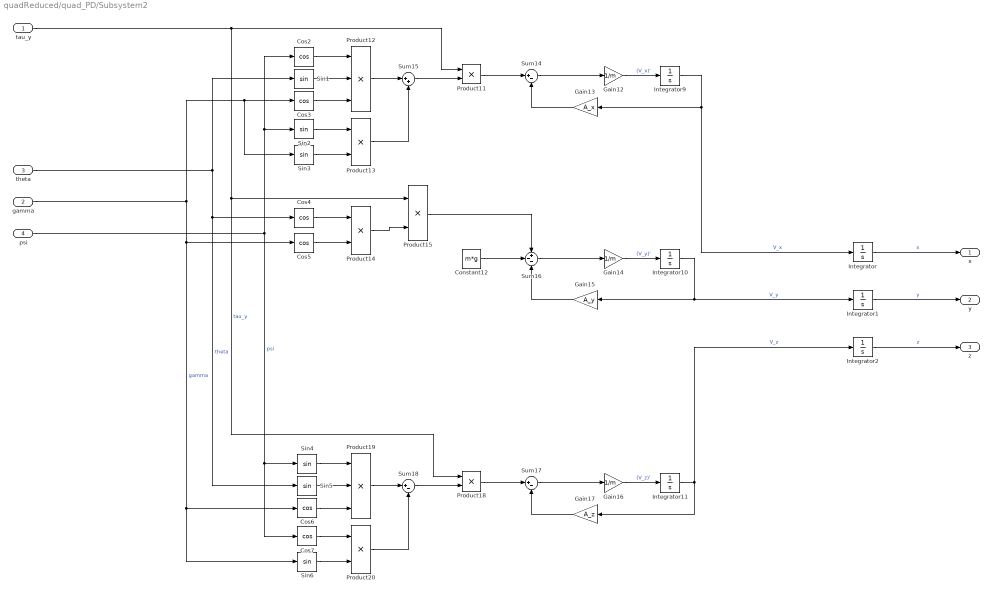
== system quadReduced/quad_PD/Subsystem2 ==
  tau_y : Inport
  gamma : Inport  Port=2
  theta : Inport  Port=3
  psi : Inport  Port=4
  Constant12 : Constant  Value=m*g
  Cos{2..7} (6 alike) : Trigonometry  Operator=cos
  Gain12 : Gain  Gain=1/m
  Gain13 : Gain  Gain=A_x
  Gain14 : Gain  Gain=1/m
  Gain15 : Gain  Gain=A_y
  Gain16 : Gain  Gain=1/m
  Gain17 : Gain  Gain=A_z
  Integrator{,1..2,9..11} (6 alike) : Integrator
  Product{11,13..15,18,20} (6 alike) : Product
  Product12 : Product  Inputs=3
  Product19 : Product  Inputs=3
  Sin{1..6} (6 alike) : Trigonometry
  Sum14 : Sum  Inputs=|+-
  Sum15 : Sum  Inputs=|++
  Sum16 : Sum  Inputs=+--
  Sum17 : Sum  Inputs=|+-
  Sum18 : Sum  Inputs=|+-
  x : Outport
  y : Outport  Port=2
  z : Outport  Port=3
  wires:
  Cos4/1 -> Product14/1
  Product15/1 -> Sum16/1
  psi/1 -> Cos7/1, Sin4/1, Cos2/1, Sin2/1  "psi"
  Cos5/1 -> Product14/2
  Product11/1 -> Sum14/1
  Sin4/1 -> Product19/1
  Sin6/1 -> Product20/2
  Integrator11/1 -> Gain17/1, Integrator2/1  "V_z"
  Cos3/1 -> Product12/3
  Gain12/1 -> Integrator9/1  "(V_x)'"
  Gain16/1 -> Integrator11/1  "(V_z)'"
  Cos2/1 -> Product12/1
  tau_y/1 -> Product18/1, Product15/1, Product11/1  "tau_y"
  Product14/1 -> Product15/2
  gamma/1 -> Sin6/1, Cos6/1, Cos5/1, Sin3/1, Cos3/1  "gamma"
  theta/1 -> Sin5/1, Cos4/1, Sin1/1  "theta"
  Integrator9/1 -> Integrator/1, Gain13/1  "V_x"
  Product20/1 -> Sum18/2
  Product19/1 -> Sum18/1
  Gain14/1 -> Integrator10/1  "(V_y)'"
  Constant12/1 -> Sum16/2
  Cos7/1 -> Product20/1
  Gain17/1 -> Sum17/2
  Sin3/1 -> Product13/2
  Gain15/1 -> Sum16/3
  Sum16/1 -> Gain14/1
  Integrator10/1 -> Integrator1/1, Gain15/1  "V_y"
  Product12/1 -> Sum15/1
  Sin1/1 -> Product12/2
  Sum15/1 -> Product11/2
  Product13/1 -> Sum15/2
  Sum14/1 -> Gain12/1
  Product18/1 -> Sum17/1
  Sin2/1 -> Product13/1
  Gain13/1 -> Sum14/2
  Sum18/1 -> Product18/2
  Sum17/1 -> Gain16/1
  Cos6/1 -> Product19/3
  Sin5/1 -> Product19/2
  Integrator/1 -> x/1  "x"
  Integrator1/1 -> y/1  "y"
  Integrator2/1 -> z/1  "z"

== system quadReduced/quad_PD/Subsystem3 ==
  omega_1 : Inport
  omega_2 : Inport  Port=2
  omega_3 : Inport  Port=3
  omega_4 : Inport  Port=4
  Gain1 : Gain  Gain=l*k
  Gain2 : Gain  Gain=l*k
  Gain3 : Gain  Gain=b
  Gain4 : Gain  Gain=k
  Math Function{,1..5} (6 alike) : Math  Operator=square  SignedPower=on
  Mux : Mux
  Mux1 : Mux
  Sum of Elements : Sum  Inputs=+
  Sum of Elements1 : Sum  Inputs=+
  Sum1 : Sum  Inputs=|-+
  Sum2 : Sum  Inputs=|-+
  tau_gamma : Outport
  tau_theta : Outport  Port=2
  tau_psi : Outport  Port=3
  tau_y : Outport  Port=4
  wires:
  Gain1/1 -> tau_theta/1
  Sum2/1 -> Gain1/1
  Sum1/1 -> Gain2/1
  Gain2/1 -> tau_gamma/1
  Math Function/1 -> Sum1/1
  Math Function1/1 -> Sum1/2
  Math Function2/1 -> Sum2/1
  Math Function3/1 -> Sum2/2
  Mux/1 -> Math Function4/1
  Math Function4/1 -> Gain3/1
  Gain3/1 -> Sum of Elements/1
  Sum of Elements/1 -> tau_psi/1
  Sum of Elements1/1 -> tau_y/1
  Gain4/1 -> Sum of Elements1/1
  Math Function5/1 -> Gain4/1
  Mux1/1 -> Math Function5/1
  omega_2/1 -> Mux1/2, Mux/2, Math Function/1
  omega_3/1 -> Math Function3/1, Mux1/3, Mux/3
  omega_1/1 -> Math Function2/1, Mux1/1, Mux/1
  omega_4/1 -> Mux1/4, Mux/4, Math Function1/1

== system quadReduced/quad_PD/Subsystem4 ==
  omega_1 : Inport
  omega_2 : Inport  Port=2
  omega_3 : Inport  Port=3
  omega_4 : Inport  Port=4
  Gain1 : Gain  Gain=l*k
  Gain2 : Gain  Gain=l*k
  Gain3 : Gain  Gain=b
  Gain4 : Gain  Gain=k
  Math Function{,1..5} (6 alike) : Math  Operator=square  SignedPower=on
  Mux : Mux
  Mux1 : Mux
  Sum of Elements : Sum  Inputs=+
  Sum of Elements1 : Sum  Inputs=+
  Sum1 : Sum  Inputs=|-+
  Sum2 : Sum  Inputs=|-+
  tau_gamma : Outport
  tau_theta : Outport  Port=2
  tau_psi : Outport  Port=3
  tau_y : Outport  Port=4
  wires:
  Gain1/1 -> tau_theta/1
  Sum2/1 -> Gain1/1
  Sum1/1 -> Gain2/1
  Gain2/1 -> tau_gamma/1
  Math Function/1 -> Sum1/1
  Math Function1/1 -> Sum1/2
  Math Function2/1 -> Sum2/1
  Math Function3/1 -> Sum2/2
  Mux/1 -> Math Function4/1
  Math Function4/1 -> Gain3/1
  Gain3/1 -> Sum of Elements/1
  Sum of Elements/1 -> tau_psi/1
  Sum of Elements1/1 -> tau_y/1
  Gain4/1 -> Sum of Elements1/1
  Math Function5/1 -> Gain4/1
  Mux1/1 -> Math Function5/1
  omega_2/1 -> Mux1/2, Mux/2, Math Function/1
  omega_3/1 -> Math Function3/1, Mux1/3, Mux/3
  omega_1/1 -> Math Function2/1, Mux1/1, Mux/1
  omega_4/1 -> Mux1/4, Mux/4, Math Function1/1

== system quadReduced/quad_PD_linear/I*angle''=torgue ==
  tau_gamma : Inport
  tau_theta : Inport  Port=2
  tau_psi : Inport  Port=3
  Constant10 : Constant  Value=I_x
  Constant12 : Constant  Value=I_z
  Constant14 : Constant  Value=I_y
  Integrator1 : Integrator
  Integrator2 : Integrator
  Integrator6 : Integrator
  Product10 : Product  Inputs=*/
  Product8 : Product  Inputs=*/
  Product9 : Product  Inputs=*/
  omega_x : Outport
  omega_y : Outport  Port=2
  omega_z : Outport  Port=3
  wires:
  tau_gamma/1 -> Product8/1  "tau_gamma"
  Product9/1 -> Integrator2/1  "(omega_y)'"
  Integrator1/1 -> omega_x/1  "omega_x"
  Constant10/1 -> Product8/2  "I_x"
  Product8/1 -> Integrator1/1  "(omega_x)'"
  Constant12/1 -> Product9/2  "I_y"
  tau_theta/1 -> Product9/1  "tau_theta"
  Integrator2/1 -> omega_y/1  "omega_y"
  Product10/1 -> Integrator6/1  "(omega_z)'"
  tau_psi/1 -> Product10/1  "tau_psi"
  Constant14/1 -> Product10/2  "I_z"
  Integrator6/1 -> omega_z/1  "omega_z"

== system quadReduced/quad_PD_linear/PD regulator draft ==
  gamma : Inport
  theta : Inport  Port=2
  y : Inport  Port=3
  Constant : Constant  Value=g
  Constant1 : Constant  Value=K_y_D
  Constant4 : Constant  Value=K_y_P
  Constant7 : Constant  Value=m
  Cos : Trigonometry  Operator=cos
  Cos1 : Trigonometry  Operator=cos
  Derivative : Derivative
  Derivative1 : Derivative
  Product{,1,3..4} (4 alike) : Product
  Product2 : Product  Inputs=*/
  Sum : Sum  Inputs=+++
  Sum1 : Sum  Inputs=|+-
  Sum2 : Sum  Inputs=|+-
  target : Constant  Value=y_d
  target1 : Constant  Value=y_d
  tau_y : Outport
  wires:
  Product2/1 -> Product4/2
  Product4/1 -> tau_y/1  "tau_y"
  Sum/1 -> Product4/1
  gamma/1 -> Cos/1  "gamma"
  theta/1 -> Cos1/1  "theta"
  Sum2/1 -> Product1/2
  Cos1/1 -> Product3/2
  Constant7/1 -> Product2/1
  Product3/1 -> Product2/2
  target1/1 -> Sum2/1
  Derivative/1 -> Sum1/1
  Constant/1 -> Sum/2
  Derivative1/1 -> Sum1/2
  y/1 -> Derivative1/1, Sum2/2  "y"
  target/1 -> Derivative/1
  Constant4/1 -> Product1/1
  Sum1/1 -> Product/2
  Product1/1 -> Sum/3
  Constant1/1 -> Product/1
  Product/1 -> Sum/1
  Cos/1 -> Product3/1

== system quadReduced/quad_PD_linear/PD regulator gamma ==
  gamma : Inport
  (gamma)' : Inport  Port=2
  Constant : Constant  Value=I_x/I_x
  Constant1 : Constant  Value=K_gamma_D
  Constant2 : Constant  Value=gamma_d
  Constant4 : Constant  Value=K_gamma_P
  Constant5 : Constant  Value=gamma_d
  Derivative : Derivative
  Product : Product
  Product1 : Product
  Product2 : Product
  Sum : Sum  Inputs=++|
  Sum1 : Sum  Inputs=|+-
  Sum2 : Sum  Inputs=|+-
  tau_gamma : Outport
  wires:
  Sum/1 -> Product2/1
  Constant/1 -> Product2/2
  Product2/1 -> tau_gamma/1  "tau_gamma"
  Sum2/1 -> Product1/2
  (gamma)'/1 -> Sum1/2
  Constant2/1 -> Derivative/1
  Derivative/1 -> Sum1/1
  Constant5/1 -> Sum2/1
  gamma/1 -> Sum2/2
  Constant4/1 -> Product1/1
  Sum1/1 -> Product/2
  Product1/1 -> Sum/2
  Constant1/1 -> Product/1
  Product/1 -> Sum/1

== system quadReduced/quad_PD_linear/PD regulator psi ==
  psi : Inport
  (psi)' : Inport  Port=2
  Constant : Constant  Value=I_y/I_y
  Constant1 : Constant  Value=K_psi_D
  Constant2 : Constant  Value=psi_d
  Constant4 : Constant  Value=K_psi_P
  Constant5 : Constant  Value=psi_d
  Derivative : Derivative
  Product : Product
  Product1 : Product
  Product2 : Product
  Sum : Sum  Inputs=++|
  Sum1 : Sum  Inputs=|+-
  Sum2 : Sum  Inputs=|+-
  tau_psi : Outport
  wires:
  Sum/1 -> Product2/1
  Constant/1 -> Product2/2
  Product2/1 -> tau_psi/1  "tau_psi"
  Sum2/1 -> Product1/2
  (psi)'/1 -> Sum1/2
  Constant2/1 -> Derivative/1
  Derivative/1 -> Sum1/1
  Constant5/1 -> Sum2/1
  psi/1 -> Sum2/2
  Constant4/1 -> Product1/1
  Sum1/1 -> Product/2
  Product1/1 -> Sum/2
  Constant1/1 -> Product/1
  Product/1 -> Sum/1

== system quadReduced/quad_PD_linear/PD regulator theta ==
  theta : Inport
  (theta)' : Inport  Port=2
  Constant : Constant  Value=I_z/I_z
  Constant1 : Constant  Value=K_theta_D
  Constant2 : Constant  Value=theta_d
  Constant4 : Constant  Value=K_theta_P
  Constant5 : Constant  Value=theta_d
  Derivative : Derivative
  Product : Product
  Product1 : Product
  Product2 : Product
  Sum : Sum  Inputs=++|
  Sum1 : Sum  Inputs=|+-
  Sum2 : Sum  Inputs=|+-
  tau_theta : Outport
  wires:
  Sum/1 -> Product2/1
  Constant/1 -> Product2/2
  Product2/1 -> tau_theta/1  "tau_theta"
  Sum2/1 -> Product1/2
  (theta)'/1 -> Sum1/2
  Constant2/1 -> Derivative/1
  Derivative/1 -> Sum1/1
  Constant5/1 -> Sum2/1
  theta/1 -> Sum2/2
  Constant4/1 -> Product1/1
  Sum1/1 -> Product/2
  Product1/1 -> Sum/2
  Constant1/1 -> Product/1
  Product/1 -> Sum/1

== system quadReduced/quad_PD_linear/Subsystem3 ==
  omega_1 : Inport
  omega_2 : Inport  Port=2
  omega_3 : Inport  Port=3
  omega_4 : Inport  Port=4
  Gain1 : Gain  Gain=l*k
  Gain2 : Gain  Gain=l*k
  Gain3 : Gain  Gain=b
  Gain4 : Gain  Gain=k
  Math Function{,1..5} (6 alike) : Math  Operator=square  SignedPower=on
  Mux : Mux
  Mux1 : Mux
  Sum of Elements : Sum  Inputs=+
  Sum of Elements1 : Sum  Inputs=+
  Sum1 : Sum  Inputs=|-+
  Sum2 : Sum  Inputs=|-+
  tau_gamma : Outport
  tau_theta : Outport  Port=2
  tau_psi : Outport  Port=3
  tau_y : Outport  Port=4
  wires:
  omega_4/1 -> Math Function1/1, Mux/4, Mux1/4
  omega_1/1 -> Mux/1, Mux1/1, Math Function2/1
  omega_3/1 -> Mux/3, Mux1/3, Math Function3/1
  omega_2/1 -> Math Function/1, Mux/2, Mux1/2
  Mux1/1 -> Math Function5/1
  Math Function5/1 -> Gain4/1
  Gain4/1 -> Sum of Elements1/1
  Sum of Elements1/1 -> tau_y/1
  Sum of Elements/1 -> tau_psi/1
  Gain3/1 -> Sum of Elements/1
  Math Function4/1 -> Gain3/1
  Mux/1 -> Math Function4/1
  Math Function3/1 -> Sum2/2
  Math Function2/1 -> Sum2/1
  Math Function1/1 -> Sum1/2
  Math Function/1 -> Sum1/1
  Gain2/1 -> tau_gamma/1
  Sum1/1 -> Gain2/1
  Sum2/1 -> Gain1/1
  Gain1/1 -> tau_theta/1

== system quadReduced/quad_PD_linear/Subsystem4 ==
  omega_1 : Inport
  omega_2 : Inport  Port=2
  omega_3 : Inport  Port=3
  omega_4 : Inport  Port=4
  Gain1 : Gain  Gain=l*k
  Gain2 : Gain  Gain=l*k
  Gain3 : Gain  Gain=b
  Gain4 : Gain  Gain=k
  Math Function{,1..5} (6 alike) : Math  Operator=square  SignedPower=on
  Mux : Mux
  Mux1 : Mux
  Sum of Elements : Sum  Inputs=+
  Sum of Elements1 : Sum  Inputs=+
  Sum1 : Sum  Inputs=|-+
  Sum2 : Sum  Inputs=|-+
  tau_gamma : Outport
  tau_theta : Outport  Port=2
  tau_psi : Outport  Port=3
  tau_y : Outport  Port=4
  wires:
  omega_4/1 -> Math Function1/1, Mux/4, Mux1/4
  omega_1/1 -> Mux/1, Mux1/1, Math Function2/1
  omega_3/1 -> Mux/3, Mux1/3, Math Function3/1
  omega_2/1 -> Math Function/1, Mux/2, Mux1/2
  Mux1/1 -> Math Function5/1
  Math Function5/1 -> Gain4/1
  Gain4/1 -> Sum of Elements1/1
  Sum of Elements1/1 -> tau_y/1
  Sum of Elements/1 -> tau_psi/1
  Gain3/1 -> Sum of Elements/1
  Math Function4/1 -> Gain3/1
  Mux/1 -> Math Function4/1
  Math Function3/1 -> Sum2/2
  Math Function2/1 -> Sum2/1
  Math Function1/1 -> Sum1/2
  Math Function/1 -> Sum1/1
  Gain2/1 -> tau_gamma/1
  Sum1/1 -> Gain2/1
  Sum2/1 -> Gain1/1
  Gain1/1 -> tau_theta/1

== system quadReduced/quad_PD_linear/angles'=omega ==
  omega_x : Inport
  omega_y : Inport  Port=2
  omega_z : Inport  Port=3
  Integrator6 : Integrator
  Integrator7 : Integrator
  Integrator8 : Integrator
  gamma : Outport
  theta : Outport  Port=2
  psi : Outport  Port=3
  (gamma)' : Outport  Port=4
  (theta)' : Outport  Port=5
  (psi)' : Outport  Port=6
  wires:
  omega_y/1 -> Integrator7/1, (theta)'/1  "(theta)'"
  Integrator8/1 -> psi/1  "psi"
  Integrator6/1 -> gamma/1  "gamma"
  Integrator7/1 -> theta/1  "theta"
  omega_x/1 -> Integrator6/1, (gamma)'/1  "(gamma)'"
  omega_z/1 -> Integrator8/1, (psi)'/1  "(psi)'"

== system quadReduced/quad_PD_linear/position ==
  tau_y : Inport
  gamma : Inport  Port=2
  theta : Inport  Port=3
  psi : Inport  Port=4
  Constant1 : Constant  Value=m*g
  Constant12 : Constant  Value=m*g
  Cos4 : Trigonometry  Operator=cos
  Cos5 : Trigonometry  Operator=cos
  Gain1 : Gain  Gain=A_y
  Gain14 : Gain  Gain=1/m
  Gain15 : Gain  Gain=A_y
  Gain2 : Gain  Gain=1/m
  Integrator{1,3..4,10} (4 alike) : Integrator
  Product14 : Product
  Product15 : Product
  Sum1 : Sum  Inputs=+--
  Sum16 : Sum  Inputs=+--
  y : Outport
  wires:
  tau_y/1 -> Product15/1, Sum1/1  "tau_y"
  Constant1/1 -> Sum1/2
  Gain1/1 -> Sum1/3
  Sum1/1 -> Gain2/1
  Integrator3/1 -> Gain1/1, Integrator4/1  "V_y"
  Gain2/1 -> Integrator3/1  "(V_y)'"
  Cos5/1 -> Product14/2
  Integrator1/1 -> y/1  "y"
  Cos4/1 -> Product14/1
  Gain14/1 -> Integrator10/1  "(V_y)'"
  theta/1 -> Cos4/1  "theta"
  Product14/1 -> Product15/2
  gamma/1 -> Cos5/1  "gamma"
  Gain15/1 -> Sum16/3
  Integrator10/1 -> Integrator1/1, Gain15/1  "V_y"
  Sum16/1 -> Gain14/1
  Constant12/1 -> Sum16/2
  Product15/1 -> Sum16/1

== system quadReduced/quad_PID/PD regulator draft ==
  gamma : Inport
  theta : Inport  Port=2
  y : Inport  Port=3
  Constant : Constant  Value=g
  Constant1 : Constant  Value=K_y_D
  Constant4 : Constant  Value=K_y_P
  Constant7 : Constant  Value=m
  Cos : Trigonometry  Operator=cos
  Cos1 : Trigonometry  Operator=cos
  Derivative : Derivative
  Derivative1 : Derivative
  Product{,1,3..4} (4 alike) : Product
  Product2 : Product  Inputs=*/
  Sum : Sum  Inputs=+++
  Sum1 : Sum  Inputs=|+-
  Sum2 : Sum  Inputs=|+-
  target : Constant  Value=y_d
  target1 : Constant  Value=y_d
  tau_y : Outport
  wires:
  Product2/1 -> Product4/2
  Product4/1 -> tau_y/1  "tau_y"
  Sum/1 -> Product4/1
  gamma/1 -> Cos/1  "gamma"
  theta/1 -> Cos1/1  "theta"
  Sum2/1 -> Product1/2
  Cos1/1 -> Product3/2
  Constant7/1 -> Product2/1
  Product3/1 -> Product2/2
  target1/1 -> Sum2/1
  Derivative/1 -> Sum1/1
  Constant/1 -> Sum/2
  Derivative1/1 -> Sum1/2
  y/1 -> Derivative1/1, Sum2/2  "y"
  target/1 -> Derivative/1
  Constant4/1 -> Product1/1
  Sum1/1 -> Product/2
  Product1/1 -> Sum/3
  Constant1/1 -> Product/1
  Product/1 -> Sum/1
  Cos/1 -> Product3/1
